simulink model "diagrama_ascensor"  (R2015a)
settings: Solver=ode45  StartTime=0.0  StopTime=10.0  RelTol=1e-3
libraries: fuzblock x1
settings Model: Creator=IngAldair  LastModifiedBy=IngAldair

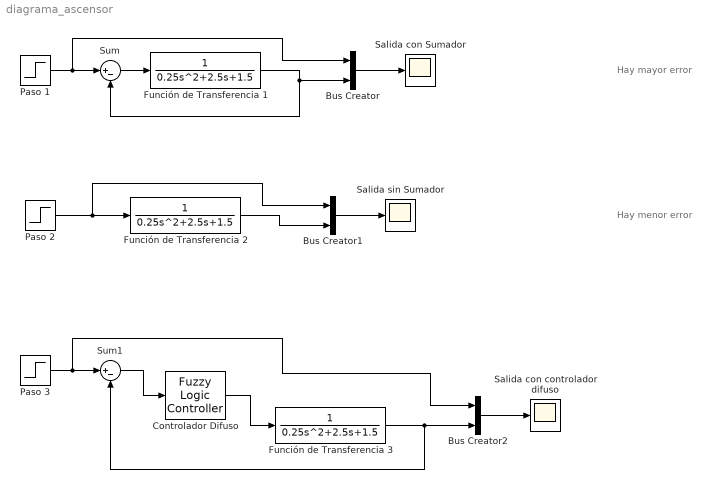
== system diagrama_ascensor ==
  note: Hay mayor error
  note: Hay menor error
  Bus Creator : BusCreator  Inputs=2
  Bus Creator1 : BusCreator  Inputs=2
  Bus Creator2 : BusCreator  Inputs=2
  Controlador Difuso : fuzblock/Fuzzy Logic  Controller  fis=controlador
  Función de Transferencia 1 : TransferFcn  Denominator=[0.25 2.5 1.5]
  Función de Transferencia 2 : TransferFcn  Denominator=[0.25 2.5 1.5]
  Función de Transferencia 3 : TransferFcn  Denominator=[0.25 2.5 1.5]
  Paso 1 : Step  SampleTime=0
  Paso 2 : Step  SampleTime=0
  Paso 3 : Step  SampleTime=0
  Salida con Sumador : Scope
      settings: TimeRange=10  YMin=0  YMax=1
  Salida con controlador difuso : Scope
      settings: TimeRange=10  YMin=0  YMax=12  SaveName=ScopeData2
  Salida sin Sumador : Scope
  Sum : Sum  Inputs=|+-
  Sum1 : Sum  Inputs=|+-
  wires:
  Bus Creator/1 -> Salida con Sumador/1
  Paso 1/1 -> Bus Creator/1, Sum/1
  Sum/1 -> Función de Transferencia 1/1
  Función de Transferencia 1/1 -> Bus Creator/2, Sum/2
  Bus Creator1/1 -> Salida sin Sumador/1
  Paso 2/1 -> Función de Transferencia 2/1, Bus Creator1/1
  Función de Transferencia 2/1 -> Bus Creator1/2
  Bus Creator2/1 -> Salida con controlador difuso/1
  Paso 3/1 -> Bus Creator2/1, Sum1/1
  Función de Transferencia 3/1 -> Bus Creator2/2, Sum1/2
  Sum1/1 -> Controlador Difuso/1
  Controlador Difuso/1 -> Función de Transferencia 3/1
